simulink library "Resettable_Derivative"  (R2020b)
settings: Solver=VariableStepAuto  StartTime=0.0  StopTime=10.0  RelTol=1e-3
undefined symbols (not defined in the file or in its folder): en_ResetStates, PauseResume
libraries: simulink x1
settings Model: Creator=matteolarcher  LastModifiedBy=matteolarcher

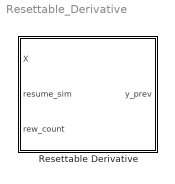
== system Resettable_Derivative ==
  Resettable Derivative : Subsystem  mask{Ts_int=0.001, X0_int=0, en_res_flag=en_ResetStates}
      mask prompts: Ts_int "sampling time"; X0_int "initial conditions"; en_res_flag "enable reset flag"

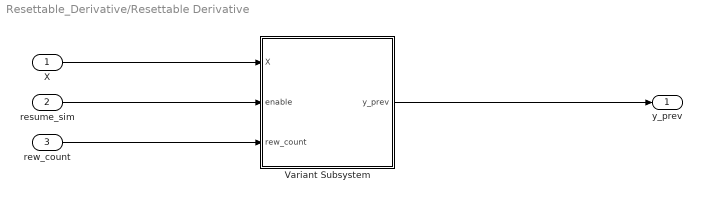
== system Resettable_Derivative/Resettable Derivative ==
  X : Inport
  resume_sim : Inport  Port=2
  rew_count : Inport  Port=3
  Variant Subsystem : Subsystem  Variant=on
  y_prev : Outport
  wires:
  X/1 -> Variant Subsystem/1(X)
  resume_sim/1 -> Variant Subsystem/2(enable)
  rew_count/1 -> Variant Subsystem/3(rew_count)
  Variant Subsystem/1(y_prev) -> y_prev/1

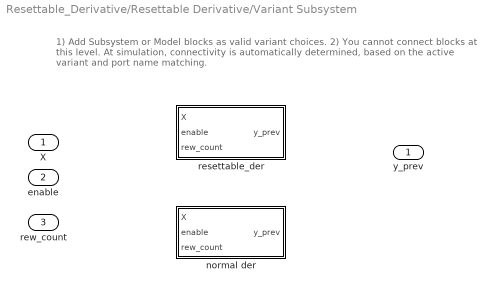
== system Resettable_Derivative/Resettable Derivative/Variant Subsystem ==
  note: 1) Add Subsystem or Model blocks as valid variant choices.
      | 2) You cannot connect blocks at this level. At simulation, connectivity is automatically
      | determined, based on the active variant and port name matching.
  X : Inport
  enable : Inport  Port=2
  rew_count : Inport  Port=3
  normal der : Subsystem  VariantControl=en_res_flag == 0
  resettable_der : Subsystem  VariantControl=en_res_flag == 1
  y_prev : Outport

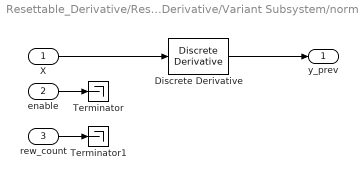
== system Resettable_Derivative/Resettable Derivative/Variant Subsystem/normal der ==
  X : Inport
  enable : Inport  Port=2
  rew_count : Inport  Port=3
  Discrete Derivative : simulink/Discrete/Discrete Derivative  gainval=1.0  ICPrevScaledInput=X0_int  OutMin=[]  OutMax=[]  OutDataType=fixdt(1, 16)  OutScaling=2^-10  DoSatur=off
  Terminator : Terminator
  Terminator1 : Terminator
  y_prev : Outport
  wires:
  enable/1 -> Terminator/1
  rew_count/1 -> Terminator1/1
  X/1 -> Discrete Derivative/1
  Discrete Derivative/1 -> y_prev/1

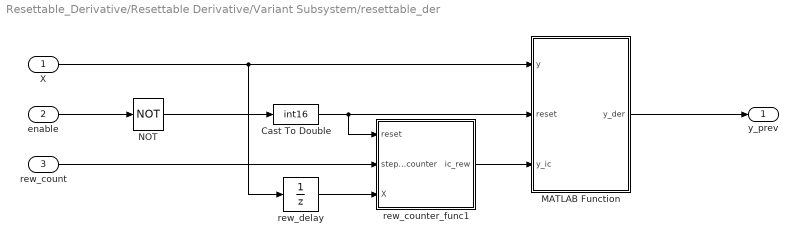
== system Resettable_Derivative/Resettable Derivative/Variant Subsystem/resettable_der ==
  X : Inport
  enable : Inport  Port=2
  rew_count : Inport  Port=3
  Cast To Double : DataTypeConversion  OutDataTypeStr=int16
  MATLAB Function : MATLAB Function  TreatAsAtomicUnit=on
  NOT : Logic  Operator=NOT  IconShape=distinctive  AllPortsSameDT=off  OutDataTypeStr=boolean
  rew_counter_func1 : MATLAB Function  TreatAsAtomicUnit=on
  rew_delay : UnitDelay  InitialCondition=X0_int  SampleTime=Ts_int  HasFrameUpgradeWarning=on
  y_prev : Outport
  wires:
  rew_delay/1 -> rew_counter_func1/3(X)
  X/1 -> rew_delay/1, MATLAB Function/1(y)
  MATLAB Function/1(y_der) -> y_prev/1
  rew_count/1 -> rew_counter_func1/2(stepback_counter)
  rew_counter_func1/1(ic_rew) -> MATLAB Function/3(y_ic)
  enable/1 -> NOT/1
  NOT/1 -> Cast To Double/1
  Cast To Double/1 -> MATLAB Function/2(reset), rew_counter_func1/1(reset)

== matlab function Resettable_Derivative/Resettable Derivative/Variant Subsystem/resettable_der/MATLAB Function ==
  data: y input; y_der output; reset input; y_ic input; Ts_int parameter
function y_der = fcn(y,reset,y_ic,Ts_int)

persistent y_store

if isempty(y_store) 
    y_store = y;
    y_der = zeros(size(y_ic));
elseif reset > 0
    y_store = y_ic;
    y_der = zeros(size(y_ic));
else
    y_der = (y-y_store)./Ts_int;
    y_store = y;
end

== matlab function Resettable_Derivative/Resettable Derivative/Variant Subsystem/resettable_der/rew_counter_func1 ==
  data: reset input; stepback_counter input size=1; X input; ic_rew output; X0_int parameter; Ts_int parameter; PauseResume parameter
%% VEHICLE REWIND STATES

function ic_rew = ic_buffer(reset, stepback_counter, X, X0_int, Ts_int, PauseResume)

persistent states_buf i reset_pre

% safety saturations
if PauseResume.rewind_time > 50
    n_states = 50;
else
    n_states = PauseResume.rewind_time;
end
if stepback_counter > n_states
    stepback_counter = int16(n_states);
end

% initialization

size_fifo = size(X0_int,2);
ic_rew = zeros(1,size_fifo);
if isempty(states_buf)
    states_buf = zeros(int16(n_states), size_fifo);
    for j=1:n_states
        states_buf(j,:) = X;
    end
end
if isempty(i)
   i = 0;
end
if isempty(reset_pre)
   reset_pre = int16(0);
end

%%%%%%%%%%

% update buffer every rewind_samp 
if mod(i,PauseResume.rewind_samp/Ts_int)==0 && reset==0 && reset_pre==0
    states_buf(2:end,:) = states_buf(1:end-1,:);
    states_buf(1,:) = X;
end

% update initial conditions
if stepback_counter > 0     % stepback resume
    ic_rew(1,:) = states_buf(stepback_counter, :);
else                        % pause-resume without stepback 
    ic_rew(1,:) = X;
end

% detect enable falling edge and update buffer
% selected
if reset_pre > reset
    remain_size = n_states-stepback_counter+1;              % number of samples older than stepback_counter to be keep
    states_buf(1:remain_size, :) = states_buf(stepback_counter:end, :);    % porto in cima alla fifo i valori rimasti del buffer più vecchi di stepback_counter
    for j=remain_size+1:n_states
        states_buf(j, :) = states_buf(remain_size, :);         % riempio la fifo con l'ultimo valore buono 
    end
end

% increase counter
i = i+1;
reset_pre = reset;
     
end
